simulink model "MODEL_FULL_SYSTEM"  (Simulink 7.8)
settings: Solver=ode1  StartTime=0.0  StopTime=inf  FixedStep=Ts  MaxStep=1e-3  RelTol=1e-3
PostLoadFcn:
  | Ts=80e-6; relays_settings_init;
InitFcn:
  | Ts=80e-6; relays_settings_init;
values from neighbouring files (symbols this model uses):
  relay_sets = xlsread('relay_settings_10272015.xlsx')    [relays_settings_init.m]
undefined symbols (not defined in the file or in its folder): dfilt, DiscIntNeverNeededParam, fdesignblkfcn, gcbh, Left, opmodbus_cb, ph, Right, type, V, X
libraries: simulink x72, modbus_lib x40, cables_lib x36, rtio_opalrt_common x21, rtlab x20, transformer_lib x13, dynamic_load_lib x12, powerlib x6, simulink_extras x6, ssn_lib x5, discretizing x4, rteventslib x4
(part 1 of 7)
settings Model: ARTEMISmethode_block_infos=$$__separator__$$MODEL_FULL_SYSTEM/ARTEMIS Guide$$__separator__$$  Creator=RE25624  LastModifiedBy=ma25949  BufferReuse=off
settings SolverCC: ZeroCrossAlgorithm=Adaptive
settings DataIOCC: ExternalInput=getinputstruct(op_snapshot1)  InitialState=getstatestruct(op_snapshot1)  LimitDataPoints=off  MaxDataPoints=90060  SignalLoggingSaveFormat=Dataset  SaveOutput=off  SignalLogging=off  DSMLogging=off  SaveTime=off  OutputSaveName=result
settings OptimizationCC: BlockReduction=off  OptimizeBlockIOStorage=off  BufferReuse=off  ExpressionFolding=off  LocalBlockOutputs=off
settings DebuggingCC: MaxConsecutiveZCsMsg=warning  IgnoredZcDiagnostic=none  SolverPrmCheckMsg=none  MultiTaskRateTransMsg=warning  FrameProcessingCompatibilityMsg=error  ModelReferenceExtraNoncontSigs=warning  StrictBusMsg=None
settings ModelReferenceCC: UpdateModelReferenceTargets=IfOutOfDate
settings SFSimCC: SFSimEcho=off
settings GRTTargetCC: TargetFunctionLibrary=C89/C90 (ANSI)

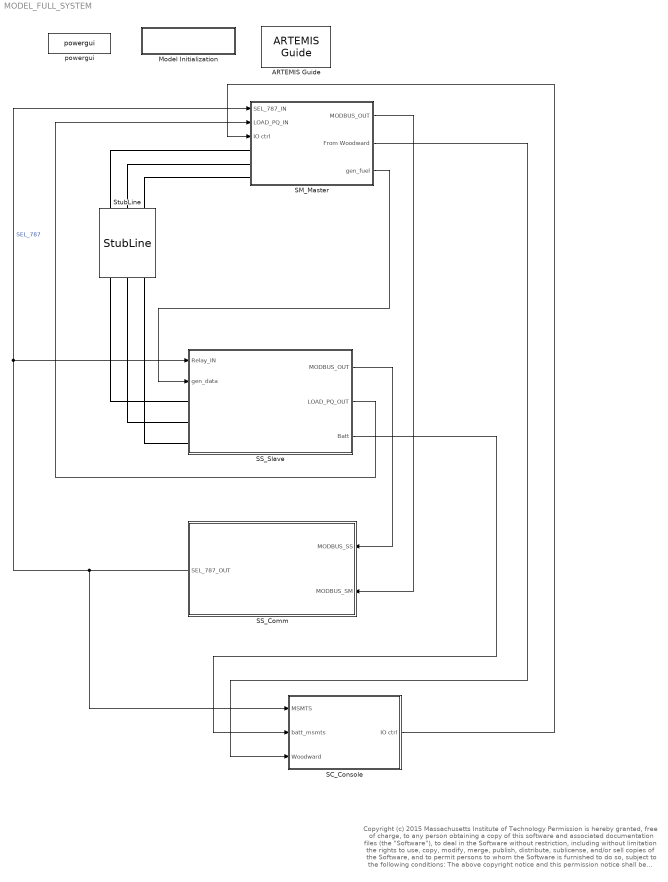
== system MODEL_FULL_SYSTEM ==
  note: Copyright (c) 2015 Massachusetts Institute of Technology
      | Permission is hereby granted, free of charge, to any person obtaining a copy of this software and associated documentation files (the "Software"), to deal in the Software without restriction, including without limitation the rights to use, copy, modify, merge, publish, distribute, sublicense, and/or sell copies of the Software, and to permit persons to whom the Software is furnished to do so, subject to the following conditions:
      |
      | The above copyright notice and this permission notice shall be included in all copies or substantial portions of the Software.
      |
      | THE SOFTWARE IS PROVIDED "AS IS", WITHOUT WARRANTY OF ANY KIND, EXPRESS OR IMPLIED, INCLUDING BUT NOT LIMITED TO THE WARRANTIES OF MERCHANTABILITY, FITNESS FOR A PARTICULAR PURPOSE AND NONINFRINGEMENT. IN NO EVENT SHALL THE AUTHORS OR COPYRIGHT HOLDERS BE LIABLE FOR ANY CLAIM,
      | DAMAGES OR OTHER LIABILITY, WHETHER IN AN ACTION OF CONTRACT, TORT OR OTHERWISE, ARISING FROM, OUT OF OR IN CONNECTION WITH THE SOFTWARE OR THE USE OR OTHER DEALINGS IN THE SOFTWARE.
  ARTEMIS Guide : artemis/ARTEMIS/ARTEMIS Guide  Tag=FTSSmethode_opal_4hx0r99  Description=5.0_z1  lock=on  Ts=Ts  opt=art5  dyna=off  nb_perm=4  RT_fullcomp=off  ssn=on  ssn_itvc=off  ssn_ivic=off  ssn_ext=off  ssn_solver=Art5 with Backward Euler nodal interface  ssn_impulse=off  ssn_quasimpulse=off  ssn_impulse_loop=2  paraExtinctionThy=off  Thy_Impulse=on  dtc=Off  dtc_opt=normal  ao=on  simtype=off  ct_mac=off  lin_mov=off  lsp=[0.001 2]  spike_skip=Disabled  dtc_extra=1  dtc_sws=normal  dtc_pied=0.5  SPSRulesBlock=SPSRules  tre=on  ctmm=off  LF=off  dpl_type=ARTEMiS DPL  rlc_type=off  custom_type=off  para=on  ssn_ImpulseLoopBlockedStateUpdate=2  ssn_mov_iter_number=5  ssn_switch_iter_number=5
  Model Initialization : Subsystem  AncestorBlock=artemis/Tools /Misc/Model Initialization  mask(Model Functions){InitFcnX=Ts=80e-6; relays_settings_init;, prel=off, posl=on, inif=on, strf=off}
      mask prompts: InitFcnX "Initialisation"; prel "Preload Function"; posl "PostLoad Function"; inif "InitFcn"; strf "StartFcn"
      mask init:
      | currentBlock = gcb;
      | root = bdroot(currentBlock);
      | 
      | if ~strcmp(get_param(root,'BlockDiagramType'),'library')
      |     if prel==1
      |         set_param(root, 'PreLoadFcn', InitFcnX);
      |     else
      |         set_param(root, 'PreLoadFcn', '');
      |     end
      |     if inif==1
      |         set_param(root, 'InitFcn', InitFcnX);
      |     else
      |         set_param(root, 'InitFcn', '');
      |     end
      |     if strf==1
      |         set_param(root, 'StartFcn', InitFcnX);
      |     else
      |         set_param(root, 'StartFcn', '');
      |     end
      |     if posl==1
      |         set_param(root, 'PostLoadFcn', InitFcnX);
      |     else
      |         set_param(root, 'PostLoadFcn', '');
      |     end
      | end
      | 
      | pos = get_param(currentBlock, 'Position');
      | width = pos(3) - pos(1); height = pos(4) - pos(2);
      | txt = [ upper(root) '\n' '- InitFcn. . . . . '  get_param(root, 'InitFcn') ];
      settings: CopyFcn=set_param(gcb,'LinkStatus','inactive')
      mask Display: text(5, height*0.5, txt, 'horizontalAlignment', 'left', 'verticalAlignment', 'middle') ;
  SC_Console : Subsystem
  SM_Master : Subsystem
  SS_Comm : Subsystem
  SS_Slave : Subsystem
  StubLine : artemis/ARTEMIS/StubLine  Phases=3  pu=on  L=1.2599e-004  Lpu=0.0475  R=0.0042  Rpu=0.002  S_base=3750E3/3  V_base=4160/sqrt(3)  F_base=60  Ts=80e-6
  powergui : powerlib/powergui  Priority=2  SimulationMode=Discrete  SolverType=Tustin  SampleTime=Ts  frequency=60  SPID=off  DisableSnubberDevices=off  DisableRonSwitches=off  DisableVfSwitches=off  SwTol=0  Interpol=off  DisplayEquations=off  FunctionMessages=off  frequencyindice=0  Pbase=100e6  ErrMax=1e-4  Iterations=50  UnitsV=kV  UnitsW=MW  echomessages=off  HookPort=off  EnableUseOfTLC=off  x0status=blocks  RestoreLinks=warning  ResistiveCurrentMeasurement=off  Frange=logspace(0,3,50)  Ylog=off  Xlog=off  ShowGrid=off  save=off  variable=ZData  structure=0  ZoomFFT=on  StartTime=0.0  cycles=2  DisplayStyle=off  fundamental=60  FreqAxis=off  MaxFrequency=1000  frequencyindicesteady=1  RmsSteady=1  display=off  Ts=0  methode=off
  wires:
  SS_Comm/1(SEL_787_OUT) -> SC_Console/1(MSMTS), SM_Master/1(SEL_787_IN), SS_Slave/1(Relay_IN)  "SEL_787"
  SM_Master/1(MODBUS_OUT) -> SS_Comm/2(MODBUS_SM)
  SS_Slave/1(MODBUS_OUT) -> SS_Comm/1(MODBUS_SS)
  SS_Slave/2(LOAD_PQ_OUT) -> SM_Master/2(LOAD_PQ_IN)
  SS_Slave/3(Batt) -> SC_Console/2(batt_msmts)
  SC_Console/1(IO ctrl) -> SM_Master/3(IO ctrl)
  SM_Master/2(From Woodward) -> SC_Console/3(Woodward)
  SM_Master/3(gen_fuel) -> SS_Slave/2(gen_data)
  connections:
  StubLine/RConn3 -- SS_Slave/LConn3
  StubLine/RConn2 -- SS_Slave/LConn2
  StubLine/RConn1 -- SS_Slave/LConn1
  StubLine/LConn3 -- SM_Master/LConn3
  StubLine/LConn2 -- SM_Master/LConn2
  StubLine/LConn1 -- SM_Master/LConn1

== system MODEL_FULL_SYSTEM/Model Initialization ==

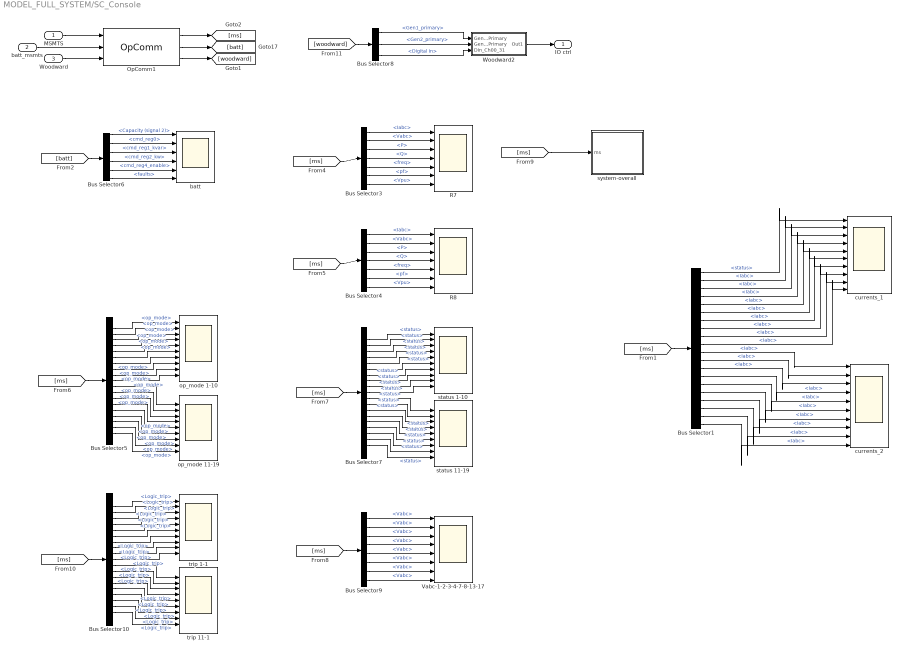
== system MODEL_FULL_SYSTEM/SC_Console ==
  MSMTS : Inport
  batt_msmts : Inport  Port=2
  Woodward : Inport  Port=3
  Bus Selector1 : BusSelector  OutputSignals=SEL_787_Relay1.m.status,SEL_787_Relay1.m.Iabc,SEL_787_Relay2.m.Iabc,SEL_787_Relay3.m.Iabc,SEL_787_Relay4.m.Iabc,SEL_787_Relay5.m.Iabc,SEL_787_Relay6.m.Iabc,SEL_787_Relay7.m.Iabc,SEL_787_Relay8.m.Iabc,SEL_787_Relay9.m.Iabc,SEL_787_Relay10.m.Iabc,SEL_787_Relay11.m.Iabc,SEL_787_Relay12.m.Iabc,SEL_787_Relay13.m.Iabc,SEL_787_Relay14.m.Iabc,SEL_787_Relay15.m.Iabc,SEL_787_Relay16.m.Iabc,SEL_787_Relay17.m.Iabc,SEL_787_Relay18.m.Iabc,SEL_787_Relay19.m.Iabc
  Bus Selector10 : BusSelector  OutputSignals=SEL_787_Relay1.Logic_trip,SEL_787_Relay2.Logic_trip,SEL_787_Relay3.Logic_trip,SEL_787_Relay4.Logic_trip,SEL_787_Relay5.Logic_trip,SEL_787_Relay6.Logic_trip,SEL_787_Relay7.Logic_trip,SEL_787_Relay8.Logic_trip,SEL_787_Relay9.Logic_trip,SEL_787_Relay10.Logic_trip,SEL_787_Relay11.Logic_trip,SEL_787_Relay12.Logic_trip,SEL_787_Relay13.Logic_trip,SEL_787_Relay14.Logic_trip,SEL_787_Relay15.Logic_trip,SEL_787_Relay16.Logic_trip,SEL_787_Relay17.Logic_trip,SEL_787_Relay18.Logic_trip,SEL_787_Relay19.Logic_trip
  Bus Selector3 : BusSelector  OutputSignals=SEL_787_Relay7.m.Iabc,SEL_787_Relay7.m.Vabc,SEL_787_Relay7.m.P,SEL_787_Relay7.m.Q,SEL_787_Relay7.m.freq,SEL_787_Relay7.m.pf,SEL_787_Relay7.m.Vpu
  Bus Selector4 : BusSelector  OutputSignals=SEL_787_Relay8.m.Iabc,SEL_787_Relay8.m.Vabc,SEL_787_Relay8.m.P,SEL_787_Relay8.m.Q,SEL_787_Relay8.m.freq,SEL_787_Relay8.m.pf,SEL_787_Relay8.m.Vpu
  Bus Selector5 : BusSelector  OutputSignals=SEL_787_Relay1.op_mode,SEL_787_Relay2.op_mode,SEL_787_Relay3.op_mode,SEL_787_Relay4.op_mode,SEL_787_Relay5.op_mode,SEL_787_Relay6.op_mode,SEL_787_Relay7.op_mode,SEL_787_Relay8.op_mode,SEL_787_Relay9.op_mode,SEL_787_Relay10.op_mode,SEL_787_Relay11.op_mode,SEL_787_Relay12.op_mode,SEL_787_Relay13.op_mode,SEL_787_Relay14.op_mode,SEL_787_Relay15.op_mode,SEL_787_Relay16.op_mode,SEL_787_Relay17.op_mode,SEL_787_Relay18.op_mode,SEL_787_Relay19.op_mode
  Bus Selector6 : BusSelector  OutputSignals=Capacity.Capacity (signal 2),controller_cmds.cmd_reg0,controller_cmds.cmd_reg1_kvar,controller_cmds.cmd_reg2_kw,controller_cmds.cmd_reg4_enable,faults
  Bus Selector7 : BusSelector  OutputSignals=SEL_787_Relay1.m.status,SEL_787_Relay2.m.status,SEL_787_Relay3.m.status,SEL_787_Relay4.m.status,SEL_787_Relay5.m.status,SEL_787_Relay6.m.status,SEL_787_Relay7.m.status,SEL_787_Relay8.m.status,SEL_787_Relay9.m.status,SEL_787_Relay10.m.status,SEL_787_Relay11.m.status,SEL_787_Relay12.m.status,SEL_787_Relay13.m.status,SEL_787_Relay14.m.status,SEL_787_Relay15.m.status,SEL_787_Relay16.m.status,SEL_787_Relay17.m.status,SEL_787_Relay18.m.status,SEL_787_Relay19.m.status
  Bus Selector8 : BusSelector  OutputSignals=Gen1_primary,Gen2_primary,Digital In
  Bus Selector9 : BusSelector  OutputSignals=SEL_787_Relay1.m.Vabc,SEL_787_Relay2.m.Vabc,SEL_787_Relay3.m.Vabc,SEL_787_Relay4.m.Vabc,SEL_787_Relay7.m.Vabc,SEL_787_Relay8.m.Vabc,SEL_787_Relay13.m.Vabc,SEL_787_Relay17.m.Vabc
  OpComm1 : rtlab/OpComm  nbport=3  groupe_acq=1  subsys_rate=0  st=0  Synchronization=on  Interpolation=on  Threshold=1.0  Missed_Data=off  Sim_Time=off  Samples=off  dynSigOut=off  from_console=0  warning_done=off  writeOpCommFile=off  Offset=off
  R7 : Scope  NumInputPorts=7
      settings: TimeRange=9  YMin=-10000~-4000~-2000000~-1000000~0~-1~0  YMax=10000~4000~2000000~3000000~80~1~2.5  SaveName=ScopeData6
  R8 : Scope  NumInputPorts=7
      settings: TimeRange=9  YMin=-1500~-150000~-10000000~-5000000~0~-1~0  YMax=1000~100000~10000000~15000000~80~1~4  SaveName=ScopeData7
  Vabc-1-2-3-4-7-8-13-17 : Scope  NumInputPorts=8
      settings: TimeRange=0.5  YMin=-1.25e+006~-40000~-40000~-40000~-750~-40000~-7500~-7500  YMax=750000~40000~40000~40000~750~40000~7500~7500  SaveName=ScopeData13
  Woodward2 : Subsystem
  batt : Scope  NumInputPorts=6
      settings: TimeRange=60  YMin=-0.5~-1~-4000~-4000~-1~-1  YMax=1.5~1~4000~4000~1~1
  currents_1 : Scope  NumInputPorts=10
      settings: TimeRange=1  YMin=0~-1000~-500~-500~-75~-300~-150~-0.0001~-0.003~-40  YMax=3~1000~500~400~75~400~200~0.0001~0.003~50  SaveName=ScopeData2
  currents_2 : Scope  NumInputPorts=10
      settings: TimeRange=1  YMin=-20~-50~-400~-300~-750~-400~-75~-750~-300~-300  YMax=25~50~400~300~750~300~75~750~300~400  SaveName=ScopeData5
  op_mode 1-10 : Scope  NumInputPorts=10
      settings: TimeRange=9  YMin=-1~-1~-1~-1~-1~-1~-1~-1~-1~-1  YMax=1~1~1~1~1~1~1~1~1~1  SaveName=ScopeData8
  op_mode 11-19 : Scope  NumInputPorts=9
      settings: TimeRange=9  YMin=-1~-1~-1~-1~-1~-1~-1~-1~-1  YMax=1~1~1~1~1~1~1~1~1  SaveName=ScopeData12
  status 1-10 : Scope  NumInputPorts=10
      settings: TimeRange=0.1  YMin=2.9999999996~2.9999999996~2.9999999996~2.9999999996~2.9999999996~2.9999999996~2.9999999996~2.9999999996~2.9999999996~2.9999999996  YMax=3.0000000004~3.0000000004~3.0000000004~3.0000000004~3.0000000004~3.0000000004~3.0000000004~3.0000000004~3.0000000004~3.0000000004  SaveName=ScopeData9
  status 11-19 : Scope  NumInputPorts=9
      settings: TimeRange=0.1  YMin=2.9999999996~2.9999999996~2.9999999996~2.9999999996~2.9999999996~2.9999999996~2.9999999996~2.9999999996~2.9999999996  YMax=3.0000000004~3.0000000004~3.0000000004~3.0000000004~3.0000000004~3.0000000004~3.0000000004~3.0000000004~3.0000000004  SaveName=ScopeData11
  system-overall : Subsystem
  trip 1-1 : Scope  NumInputPorts=10
      settings: TimeRange=9  YMin=0~0~0~0~0~0~0~0~0~0  YMax=2~2~2~2~2~2~2~2~2~2  SaveName=ScopeData15
  trip 11-1 : Scope  NumInputPorts=9
      settings: TimeRange=9  YMin=0~0~0~0~0~0~0~0~0  YMax=2~2~2~2~2~2~2~2~2  SaveName=ScopeData16
  IO ctrl : Outport
  wires:
  MSMTS/1 -> OpComm1/1
  batt_msmts/1 -> OpComm1/2
  OpComm1/2 -> [batt]
  Woodward/1 -> OpComm1/3
  OpComm1/3 -> [woodward]
  Woodward2/1(Out1) -> IO ctrl/1
  [woodward] -> Bus Selector8/1
  Bus Selector8/1 -> Woodward2/1(Gen1_Primary)  "<Gen1_primary>"
  Bus Selector8/2 -> Woodward2/2(Gen2_Primary)  "<Gen2_primary>"
  Bus Selector8/3 -> Woodward2/3(DIn_Ch00_31)  "<Digital In>"
  OpComm1/1 -> [ms]
  Bus Selector6/1 -> batt/1  "<Capacity (signal 2)>"
  Bus Selector6/2 -> batt/2  "<cmd_reg0>"
  Bus Selector6/3 -> batt/3  "<cmd_reg1_kvar>"
  Bus Selector6/4 -> batt/4  "<cmd_reg2_kw>"
  Bus Selector6/5 -> batt/5  "<cmd_reg4_enable>"
  Bus Selector6/6 -> batt/6  "<faults>"
  [batt] -> Bus Selector6/1
  [ms] -> Bus Selector1/1
  [ms] -> Bus Selector3/1
  [ms] -> Bus Selector4/1
  [ms] -> Bus Selector5/1
  [ms] -> Bus Selector7/1
  [ms] -> Bus Selector9/1
  Bus Selector5/1 -> op_mode 1-10/1  "<op_mode>"
  Bus Selector5/2 -> op_mode 1-10/2  "<op_mode>"
  Bus Selector5/3 -> op_mode 1-10/3  "<op_mode>"
  Bus Selector5/4 -> op_mode 1-10/4  "<op_mode>"
  Bus Selector5/5 -> op_mode 1-10/5  "<op_mode>"
  Bus Selector5/6 -> op_mode 1-10/6  "<op_mode>"
  Bus Selector5/7 -> op_mode 1-10/7  "<op_mode>"
  Bus Selector5/8 -> op_mode 1-10/8  "<op_mode>"
  Bus Selector5/9 -> op_mode 1-10/9  "<op_mode>"
  Bus Selector5/10 -> op_mode 1-10/10  "<op_mode>"
  Bus Selector7/1 -> status 1-10/1  "<status>"
  Bus Selector7/2 -> status 1-10/2  "<status>"
  Bus Selector7/3 -> status 1-10/3  "<status>"
  Bus Selector7/4 -> status 1-10/4  "<status>"
  Bus Selector7/5 -> status 1-10/5  "<status>"
  Bus Selector7/6 -> status 1-10/6  "<status>"
  Bus Selector7/7 -> status 1-10/7  "<status>"
  Bus Selector7/8 -> status 1-10/8  "<status>"
  Bus Selector7/9 -> status 1-10/9  "<status>"
  Bus Selector7/10 -> status 1-10/10  "<status>"
  Bus Selector5/11 -> op_mode 11-19/1  "<op_mode>"
  Bus Selector5/12 -> op_mode 11-19/2  "<op_mode>"
  Bus Selector5/13 -> op_mode 11-19/3  "<op_mode>"
  Bus Selector5/14 -> op_mode 11-19/4  "<op_mode>"
  Bus Selector5/15 -> op_mode 11-19/5  "<op_mode>"
  Bus Selector5/16 -> op_mode 11-19/6  "<op_mode>"
  Bus Selector5/17 -> op_mode 11-19/7  "<op_mode>"
  Bus Selector5/18 -> op_mode 11-19/8  "<op_mode>"
  Bus Selector5/19 -> op_mode 11-19/9  "<op_mode>"
  Bus Selector7/11 -> status 11-19/1  "<status>"
  Bus Selector7/12 -> status 11-19/2  "<status>"
  Bus Selector7/13 -> status 11-19/3  "<status>"
  Bus Selector7/14 -> status 11-19/4  "<status>"
  Bus Selector7/15 -> status 11-19/5  "<status>"
  Bus Selector7/16 -> status 11-19/6  "<status>"
  Bus Selector7/17 -> status 11-19/7  "<status>"
  Bus Selector7/18 -> status 11-19/8  "<status>"
  Bus Selector7/19 -> status 11-19/9  "<status>"
  Bus Selector3/1 -> R7/1  "<Iabc>"
  Bus Selector3/2 -> R7/2  "<Vabc>"
  Bus Selector3/3 -> R7/3  "<P>"
  Bus Selector3/4 -> R7/4  "<Q>"
  Bus Selector3/5 -> R7/5  "<freq>"
  Bus Selector3/6 -> R7/6  "<pf>"
  Bus Selector3/7 -> R7/7  "<Vpu>"
  Bus Selector4/1 -> R8/1  "<Iabc>"
  Bus Selector4/2 -> R8/2  "<Vabc>"
  Bus Selector4/3 -> R8/3  "<P>"
  Bus Selector4/4 -> R8/4  "<Q>"
  Bus Selector4/5 -> R8/5  "<freq>"
  Bus Selector4/6 -> R8/6  "<pf>"
  Bus Selector4/7 -> R8/7  "<Vpu>"
  [ms] -> system-overall/1(ms)
  [ms] -> Bus Selector10/1
  Bus Selector10/1 -> trip 1-1/1  "<Logic_trip>"
  Bus Selector10/2 -> trip 1-1/2  "<Logic_trip>"
  Bus Selector10/3 -> trip 1-1/3  "<Logic_trip>"
  Bus Selector10/4 -> trip 1-1/4  "<Logic_trip>"
  Bus Selector10/5 -> trip 1-1/5  "<Logic_trip>"
  Bus Selector10/6 -> trip 1-1/6  "<Logic_trip>"
  Bus Selector10/7 -> trip 1-1/7  "<Logic_trip>"
  Bus Selector10/8 -> trip 1-1/8  "<Logic_trip>"
  Bus Selector10/9 -> trip 1-1/9  "<Logic_trip>"
  Bus Selector10/10 -> trip 1-1/10  "<Logic_trip>"
  Bus Selector10/11 -> trip 11-1/1  "<Logic_trip>"
  Bus Selector10/12 -> trip 11-1/2  "<Logic_trip>"
  Bus Selector10/13 -> trip 11-1/3  "<Logic_trip>"
  Bus Selector10/14 -> trip 11-1/4  "<Logic_trip>"
  Bus Selector10/15 -> trip 11-1/5  "<Logic_trip>"
  Bus Selector10/16 -> trip 11-1/6  "<Logic_trip>"
  Bus Selector10/17 -> trip 11-1/7  "<Logic_trip>"
  Bus Selector10/18 -> trip 11-1/8  "<Logic_trip>"
  Bus Selector10/19 -> trip 11-1/9  "<Logic_trip>"
  Bus Selector9/1 -> Vabc-1-2-3-4-7-8-13-17/1  "<Vabc>"
  Bus Selector9/2 -> Vabc-1-2-3-4-7-8-13-17/2  "<Vabc>"
  Bus Selector9/3 -> Vabc-1-2-3-4-7-8-13-17/3  "<Vabc>"
  Bus Selector9/4 -> Vabc-1-2-3-4-7-8-13-17/4  "<Vabc>"
  Bus Selector9/5 -> Vabc-1-2-3-4-7-8-13-17/5  "<Vabc>"
  Bus Selector9/6 -> Vabc-1-2-3-4-7-8-13-17/6  "<Vabc>"
  Bus Selector9/7 -> Vabc-1-2-3-4-7-8-13-17/7  "<Vabc>"
  Bus Selector9/8 -> Vabc-1-2-3-4-7-8-13-17/8  "<Vabc>"
  Bus Selector1/1 -> currents_1/1  "<status>"
  Bus Selector1/2 -> currents_1/2  "<Iabc>"
  Bus Selector1/3 -> currents_1/3  "<Iabc>"
  Bus Selector1/4 -> currents_1/4  "<Iabc>"
  Bus Selector1/5 -> currents_1/5  "<Iabc>"
  Bus Selector1/6 -> currents_1/6  "<Iabc>"
  Bus Selector1/7 -> currents_1/7  "<Iabc>"
  Bus Selector1/8 -> currents_1/8  "<Iabc>"
  Bus Selector1/9 -> currents_1/9  "<Iabc>"
  Bus Selector1/10 -> currents_1/10  "<Iabc>"
  Bus Selector1/11 -> currents_2/1  "<Iabc>"
  Bus Selector1/12 -> currents_2/2  "<Iabc>"
  Bus Selector1/13 -> currents_2/3  "<Iabc>"
  Bus Selector1/14 -> currents_2/4  "<Iabc>"
  Bus Selector1/15 -> currents_2/5  "<Iabc>"
  Bus Selector1/16 -> currents_2/6  "<Iabc>"
  Bus Selector1/17 -> currents_2/7  "<Iabc>"
  Bus Selector1/18 -> currents_2/8  "<Iabc>"
  Bus Selector1/19 -> currents_2/9  "<Iabc>"
  Bus Selector1/20 -> currents_2/10  "<Iabc>"
